simulink model "readData"  (R2022a)
settings: Solver=FixedStepAuto  StartTime=0.0  StopTime=10  FixedStep=1/2000  RelTol=1e-3
undefined symbols (not defined in the file): communication_rate
settings Model: Creator=Mechatronics  LastModifiedBy=Mechatronics

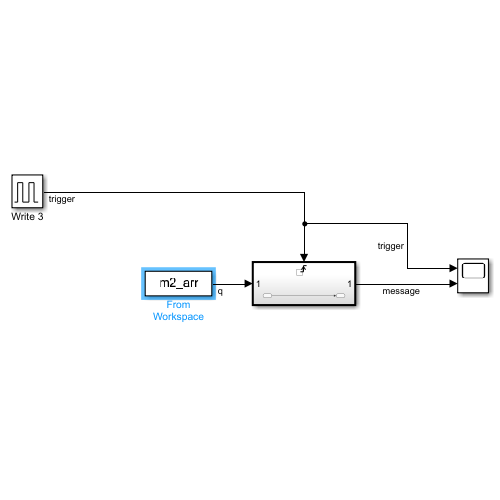
[thumbnail: Simulink's stored preview of the top-level diagram]
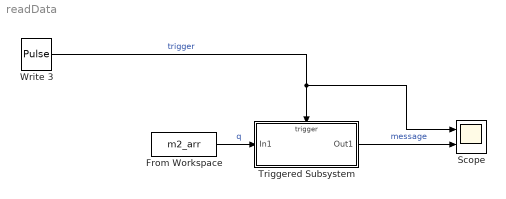
== system readData ==
  From Workspace : FromWorkspace  VariableName=m2_arr  SampleTime=-1  OutputAfterFinalValue=Holding final value
  Scope : Scope  NumInputPorts=2
  Triggered Subsystem : Subsystem  TreatAsAtomicUnit=on
  Write 3 : DiscretePulseGenerator  PulseType=Time based  Period=1/communication_rate  PulseWidth=50  PhaseDelay=5
  wires:
  Write 3/1 -> Scope/1, Triggered Subsystem/Trigger  "trigger"
  From Workspace/1 -> Triggered Subsystem/1(In1)  "q"
  Triggered Subsystem/1(Out1) -> Scope/2  "message"

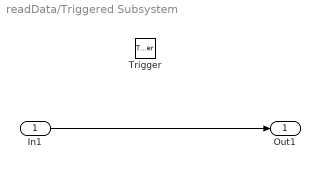
== system readData/Triggered Subsystem ==
  In1 : Inport
  Trigger : TriggerPort  VariantControl=(inherit)
  Out1 : Outport
  wires:
  In1/1 -> Out1/1
